simulink model "Dynamics"  (R2016b)
settings: Solver=FixedStepAuto  StartTime=0.0  StopTime=1.5  FixedStep=1e-3  RelTol=1e-3
values from neighbouring files (symbols this model uses):
  K = K_r(i)    [Proj_1a.m]    (also in Proj_1b.m; Proj_5.m = K_i(i))
  K_dth = 0.05    [Proj_1b.m]    (also in Proj_5.m = -0.04; parameters.m = 0.05*sgn)
  M_d = M_d_r(i)    [Proj_7.m]    (also in parameters.m = 200*sgn)
  T_m = 120    [parameters.m]
  tau = tau_i(i)    [Proj_4.m]    (also in parameters.m = 0.05)
settings Model: Creator=Daniel  LastModifiedBy=Daniel

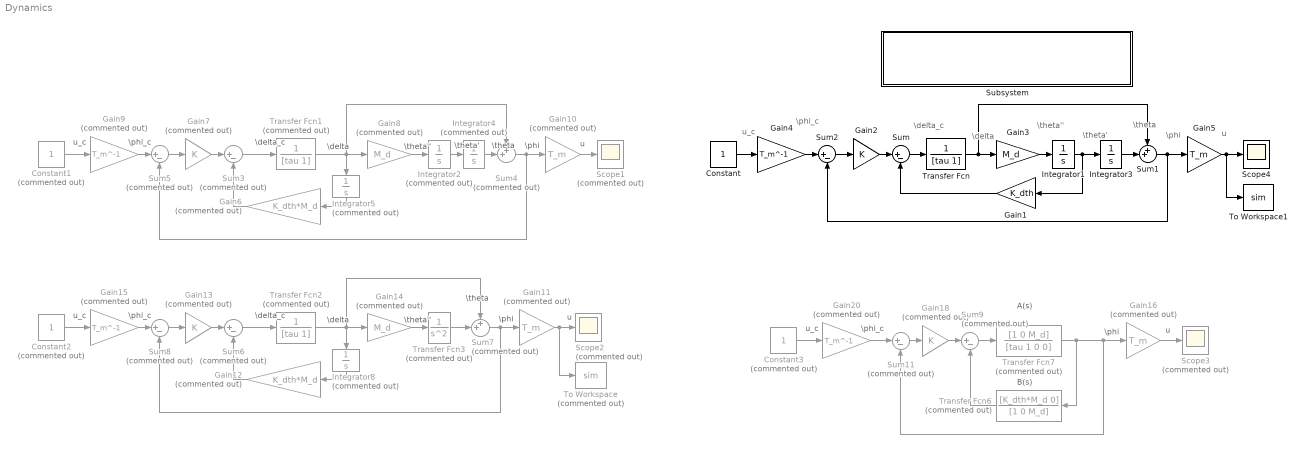
== system Dynamics ==
  note: \theta'
  note: \theta''
  note: \theta
  note: \delta
  note: \delta_c
  note: \phi_c
  note: \phi
  note: u
  note: u_c
  note: \theta''
  note: \theta
  note: \delta
  note: \delta_c
  note: \phi_c
  note: \phi
  note: u
  note: u_c
  note: \theta'
  note: \theta''
  note: \theta
  note: \delta
  note: \delta_c
  note: \phi_c
  note: \phi
  note: u
  note: u_c
  note: \phi_c
  note: \phi
  note: u
  note: u_c
  note: A(s)
  note: B(s)
  Constant : Constant
  Constant1 : Constant  Commented=on
  Constant2 : Constant  Commented=on
  Constant3 : Constant  Commented=on
  Gain1 : Gain  Gain=K_dth
  Gain10 : Gain  Commented=on  Gain=T_m
  Gain11 : Gain  Commented=on  Gain=T_m
  Gain12 : Gain  Commented=on  Gain=K_dth*M_d
  Gain13 : Gain  Commented=on  Gain=K
  Gain14 : Gain  Commented=on  Gain=M_d
  Gain15 : Gain  Commented=on  Gain=T_m^-1
  Gain16 : Gain  Commented=on  Gain=T_m
  Gain18 : Gain  Commented=on  Gain=K
  Gain2 : Gain  Gain=K
  Gain20 : Gain  Commented=on  Gain=T_m^-1
  Gain3 : Gain  Gain=M_d
  Gain4 : Gain  Gain=T_m^-1
  Gain5 : Gain  Gain=T_m
  Gain6 : Gain  Commented=on  Gain=K_dth*M_d
  Gain7 : Gain  Commented=on  Gain=K
  Gain8 : Gain  Commented=on  Gain=M_d
  Gain9 : Gain  Commented=on  Gain=T_m^-1
  Integrator1 : Integrator
  Integrator{2,4..5,8} (4 alike) : Integrator  Commented=on
  Integrator3 : Integrator
  Scope1 : Scope  Commented=on
  Scope2 : Scope  Commented=on
  Scope3 : Scope  Commented=on
  Scope4 : Scope
  Subsystem : Subsystem
      mask Display: image('Gm_s_function.PNG');
  Sum : Sum  Inputs=|+-
  Sum1 : Sum  Inputs=++|
  Sum{3,5..6,8..9,11} (6 alike) : Sum  Commented=on  Inputs=|+-
  Sum2 : Sum  Inputs=|+-
  Sum4 : Sum  Commented=on  Inputs=++|
  Sum7 : Sum  Commented=on  Inputs=++|
  To Workspace : ToWorkspace  Commented=on  VariableName=sim  SaveFormat=Timeseries  SampleTime=-1
  To Workspace1 : ToWorkspace  VariableName=sim  SaveFormat=Timeseries  SampleTime=-1
  Transfer Fcn : TransferFcn  Denominator=[tau 1]
  Transfer Fcn1 : TransferFcn  Commented=on  Denominator=[tau 1]
  Transfer Fcn2 : TransferFcn  Commented=on  Denominator=[tau 1]
  Transfer Fcn3 : TransferFcn  Commented=on  Denominator=[1 0 0]
  Transfer Fcn6 : TransferFcn  Commented=on  Numerator=[K_dth*M_d 0]  Denominator=[1 0 M_d]
  Transfer Fcn7 : TransferFcn  Commented=on  Numerator=[1 0 M_d]  Denominator=[tau 1 0 0]
  wires:
  Gain1/1 -> Sum/2
  Sum/1 -> Transfer Fcn/1
  Gain2/1 -> Sum/1
  Transfer Fcn/1 -> Sum1/1, Gain3/1
  Sum1/1 -> Sum2/2, Gain5/1
  Gain3/1 -> Integrator1/1
  Integrator1/1 -> Integrator3/1, Gain1/1
  Integrator3/1 -> Sum1/2
  Sum2/1 -> Gain2/1
  Gain5/1 -> Scope4/1, To Workspace1/1
  Constant/1 -> Gain4/1
  Gain4/1 -> Sum2/1
  Sum3/1 -> Transfer Fcn1/1
  Gain7/1 -> Sum3/1
  Transfer Fcn1/1 -> Gain8/1, Sum4/1, Integrator5/1
  Sum4/1 -> Gain10/1, Sum5/2
  Gain8/1 -> Integrator2/1
  Integrator2/1 -> Integrator4/1
  Sum5/1 -> Gain7/1
  Gain10/1 -> Scope1/1
  Constant1/1 -> Gain9/1
  Gain9/1 -> Sum5/1
  Gain6/1 -> Sum3/2
  Integrator4/1 -> Sum4/2
  Integrator5/1 -> Gain6/1
  Sum6/1 -> Transfer Fcn2/1
  Gain13/1 -> Sum6/1
  Transfer Fcn2/1 -> Integrator8/1, Sum7/1, Gain14/1
  Sum7/1 -> Sum8/2, Gain11/1
  Sum8/1 -> Gain13/1
  Gain11/1 -> To Workspace/1, Scope2/1
  Constant2/1 -> Gain15/1
  Gain15/1 -> Sum8/1
  Gain12/1 -> Sum6/2
  Transfer Fcn3/1 -> Sum7/2
  Integrator8/1 -> Gain12/1
  Gain14/1 -> Transfer Fcn3/1
  Gain18/1 -> Sum9/1
  Transfer Fcn7/1 -> Gain16/1, Sum11/2, Transfer Fcn6/1
  Sum11/1 -> Gain18/1
  Gain16/1 -> Scope3/1
  Constant3/1 -> Gain20/1
  Gain20/1 -> Sum11/1
  Sum9/1 -> Transfer Fcn7/1
  Transfer Fcn6/1 -> Sum9/2

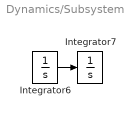
== system Dynamics/Subsystem ==
  Integrator6 : Integrator
  Integrator7 : Integrator
  wires:
  Integrator6/1 -> Integrator7/1
